simulink model "quadmanipulation"  (R2020a)
settings: Solver=VariableStepAuto  StartTime=0.0  StopTime=30  RelTol=1e-3
values from neighbouring files (symbols this model uses):
  A = [0 0 0 1 0 0 0 0 0 0 0 0 0 0 0 0 ... (first row only)    [quadmanipulation.m]
  B = [0 0 0 0 0 0 ... (first row only)    [quadmanipulation.m]
  B_imp = diag(b_imp)    [quadmanipulation.m]
  G_arm = [(m1+m2)*a1*g*cos(theta1)+m2*g*a2*cos(theta1+theta2) ... (first row only)    [quadmanipulation.m]
  JT = transpose(J)    [quadmanipulation.m]
  K_imp = diag(k_imp)    [quadmanipulation.m]
  M = [m1*a1^2+m2*(a1^2+2*a1*a2*cos(theta2)+a2^2) m2*(a1*a2*cos(theta2)+a2^2) ... (first row only)    [quadmanipulation.m]
  S_arm = [-2*m2*a1*a2*sin(theta2)*theta2_dot -m2*a1*a2*sin(theta2)*theta2_dot ... (first row only)    [quadmanipulation.m]
  theta11 = real(Theta11), theta12 = real(Theta12)    [quadmanipulation.m]
  theta21 = real(Theta21), theta22 = real(Theta22)    [quadmanipulation.m]
undefined symbols (not defined in the file or in its folder): K, theta12, theta22
settings Model: Creator=Dr.Saraf  LastModifiedBy=Dr.Saraf

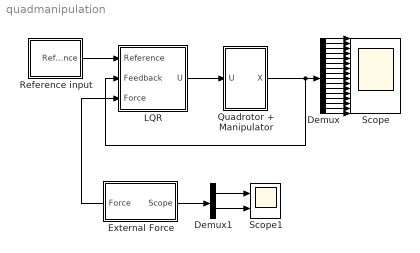
== system quadmanipulation ==
  Demux : Demux  Outputs=16
  Demux1 : Demux  Outputs=2
  External Force : Subsystem
      settings: PortSchema="{\"entries\":[{\"content\":{\"sides\":[{\"content\":{\"connectorIds\":[\"Out2\"]},\"type\":\"ConnectorPlacement.EquallySpacedRectSide\",\"uuid\":\"bc6f37bf-b6c5-4028-b4a4-1f6ac3343290\"},{\"content\":{\"connectorIds\":[\"Out1\"],\"side\":\"RIGHT\"},\"type\":\"ConnectorPlacement.EquallySpacedRectSide\",\"uuid\":\"4c1d6f8d-9a15-4436-8744-0df7d527871c\"},{\"content\":{\"connectorIds\":[],\"side\":\"TOP\"},\"type\":\"ConnectorPlacement.EquallySpacedRectSide\",\"uuid\":\"b806ddfa-c017-4b4f-bf2f-a13602b353a7\"}]},\"type\":\"ConnectorPlacement.EquallySpacedConnector\",\"uuid\":\"efa4b6a4-9e82-4f59-9dc9-02b8956516e8\"}],\"packageUris\":[\"http://schema.mathworks.com/mf0/Connector/19700101\"],\"version\":\"1.0\"}"
  LQR : Subsystem
  Quadrotor + Manipulator : Subsystem
  Reference input : Subsystem
  Scope : Scope  NumInputPorts=16
  Scope1 : Scope  NumInputPorts=2
  wires:
  Quadrotor + Manipulator/1(X) -> LQR/2(Feedback), Demux/1
  Demux/6 -> Scope/6
  Demux/1 -> Scope/1
  Demux/4 -> Scope/4
  LQR/1(U) -> Quadrotor + Manipulator/1(U)
  Demux/3 -> Scope/3
  Demux/5 -> Scope/5
  Demux/2 -> Scope/2
  Reference input/1(Reference) -> LQR/1(Reference)
  Demux/7 -> Scope/7
  Demux/8 -> Scope/8
  Demux/9 -> Scope/9
  Demux/10 -> Scope/10
  Demux/11 -> Scope/11
  Demux/12 -> Scope/12
  Demux/13 -> Scope/13
  Demux/14 -> Scope/14
  Demux/15 -> Scope/15
  Demux/16 -> Scope/16
  External Force/2(Force) -> LQR/3(Force)
  External Force/1(Scope) -> Demux1/1
  Demux1/1 -> Scope1/1
  Demux1/2 -> Scope1/2

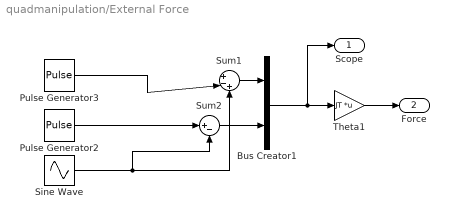
== system quadmanipulation/External Force ==
  Bus Creator1 : BusCreator  Inputs=2
  Pulse Generator2 : DiscretePulseGenerator  PulseType=Time based  Amplitude=4  Period=10  PulseWidth=20
  Pulse Generator3 : DiscretePulseGenerator  PulseType=Time based  Amplitude=5  Period=10  PulseWidth=10  PhaseDelay=4
  Sine Wave : Sin  Amplitude=2  Frequency=2  SampleTime=0
  Sum1 : Sum  Inputs=|+-+
  Sum2 : Sum  Inputs=|+-
  Theta1 : Gain  Gain=JT  Multiplication=Matrix(K*u)
  Scope : Outport
  Force : Outport  Port=2
  wires:
  Bus Creator1/1 -> Scope/1, Theta1/1
  Theta1/1 -> Force/1
  Pulse Generator3/1 -> Sum1/2
  Pulse Generator2/1 -> Sum2/1
  Sine Wave/1 -> Sum2/2, Sum1/3
  Sum2/1 -> Bus Creator1/2
  Sum1/1 -> Bus Creator1/1

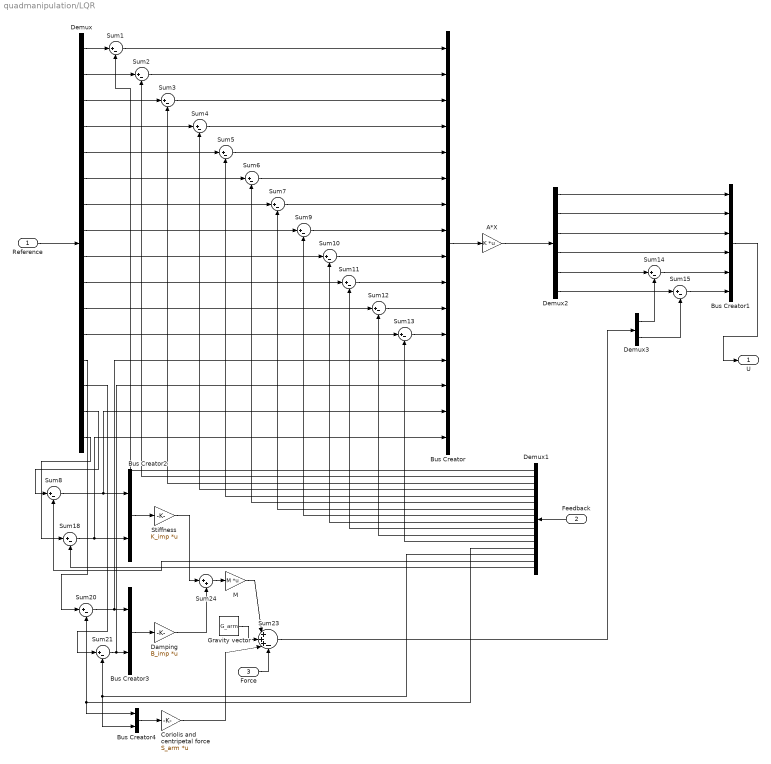
== system quadmanipulation/LQR ==
  Reference : Inport
  Feedback : Inport  Port=2
  Force : Inport  Port=3
  A*X : Gain  Gain=K  Multiplication=Matrix(K*u)
  Bus Creator : BusCreator  Inputs=16
  Bus Creator1 : BusCreator  Inputs=6
  Bus Creator2 : BusCreator  Inputs=2
  Bus Creator3 : BusCreator  Inputs=2
  Bus Creator4 : BusCreator  Inputs=2
  Coriolis and centripetal force : Gain  Gain=S_arm  Multiplication=Matrix(K*u)
  Damping : Gain  Gain=B_imp  Multiplication=Matrix(K*u)
  Demux : Demux  Outputs=16
  Demux1 : Demux  Outputs=16
  Demux2 : Demux  Outputs=6
  Demux3 : Demux  Outputs=2
  Gravity vector : Constant  Value=G_arm  VectorParams1D=off
  M : Gain  Gain=M  Multiplication=Matrix(K*u)
  Stiffness : Gain  Gain=K_imp  Multiplication=Matrix(K*u)
  Sum{1..15,18,20..21} (18 alike) : Sum  Inputs=|+-
  Sum23 : Sum  Inputs=|+++-
  Sum24 : Sum  Inputs=|++
  U : Outport
  wires:
  Bus Creator/1 -> A*X/1
  Sum2/1 -> Bus Creator/2
  Sum6/1 -> Bus Creator/6
  Sum3/1 -> Bus Creator/3
  Sum5/1 -> Bus Creator/5
  Sum4/1 -> Bus Creator/4
  Demux/6 -> Sum6/1
  Demux1/5 -> Sum5/2
  Demux1/3 -> Sum3/2
  Demux1/2 -> Sum2/2
  Demux/1 -> Sum1/1
  Sum1/1 -> Bus Creator/1
  Demux1/4 -> Sum4/2
  Demux1/6 -> Sum6/2
  Demux/2 -> Sum2/1
  Demux1/1 -> Sum1/2
  Feedback/1 -> Demux1/1
  Demux/3 -> Sum3/1
  Demux/5 -> Sum5/1
  Demux/4 -> Sum4/1
  Reference/1 -> Demux/1
  Sum13/1 -> Bus Creator/12
  Demux/12 -> Sum13/1
  Sum12/1 -> Bus Creator/11
  Demux/11 -> Sum12/1
  Sum11/1 -> Bus Creator/10
  Demux/10 -> Sum11/1
  Sum10/1 -> Bus Creator/9
  Demux/9 -> Sum10/1
  Sum9/1 -> Bus Creator/8
  Sum7/1 -> Bus Creator/7
  Demux/7 -> Sum7/1
  Demux/8 -> Sum9/1
  Demux1/7 -> Sum7/2
  Demux1/8 -> Sum9/2
  Demux1/9 -> Sum10/2
  Demux1/10 -> Sum11/2
  Demux1/11 -> Sum12/2
  Demux1/12 -> Sum13/2
  Demux/14 -> Sum21/1
  Bus Creator3/1 -> Damping/1
  Coriolis and centripetal force/1 -> Sum23/3
  Sum24/1 -> M/1
  Demux/15 -> Sum8/1
  Demux1/15 -> Sum8/2
  Sum18/1 -> Bus Creator/16, Bus Creator2/2
  Demux1/16 -> Sum18/2
  Damping/1 -> Sum24/2
  Demux/13 -> Sum20/1
  Sum20/1 -> Bus Creator/13, Bus Creator3/1
  Demux/16 -> Sum18/1
  Sum21/1 -> Bus Creator/14, Bus Creator3/2
  Force/1 -> Sum23/4
  Bus Creator4/1 -> Coriolis and centripetal force/1
  M/1 -> Sum23/1
  Bus Creator2/1 -> Stiffness/1
  Gravity vector/1 -> Sum23/2
  Stiffness/1 -> Sum24/1
  Sum8/1 -> Bus Creator/15, Bus Creator2/1
  Demux1/13 -> Bus Creator4/1, Sum20/2
  Demux1/14 -> Bus Creator4/2, Sum21/2
  Bus Creator1/1 -> U/1
  A*X/1 -> Demux2/1
  Sum23/1 -> Demux3/1
  Sum15/1 -> Bus Creator1/6
  Demux2/1 -> Bus Creator1/1
  Demux2/2 -> Bus Creator1/2
  Demux2/3 -> Bus Creator1/3
  Demux2/4 -> Bus Creator1/4
  Demux2/5 -> Sum14/1
  Sum14/1 -> Bus Creator1/5
  Demux2/6 -> Sum15/1
  Demux3/1 -> Sum14/2
  Demux3/2 -> Sum15/2

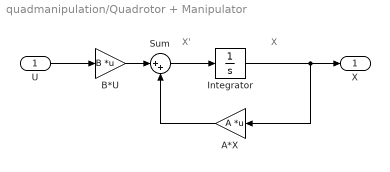
== system quadmanipulation/Quadrotor + Manipulator ==
  note: X'
  note: X
  U : Inport
  A*X : Gain  Gain=A  Multiplication=Matrix(K*u)
  B*U : Gain  Gain=B  Multiplication=Matrix(K*u)
  Integrator : Integrator  InitialCondition=[0,0,0,0,0,0,0,0,0,0,0,0,0,0,theta11, theta12]
  Sum : Sum  Inputs=|++
  X : Outport
  wires:
  Integrator/1 -> X/1, A*X/1
  Sum/1 -> Integrator/1
  U/1 -> B*U/1
  A*X/1 -> Sum/2
  B*U/1 -> Sum/1

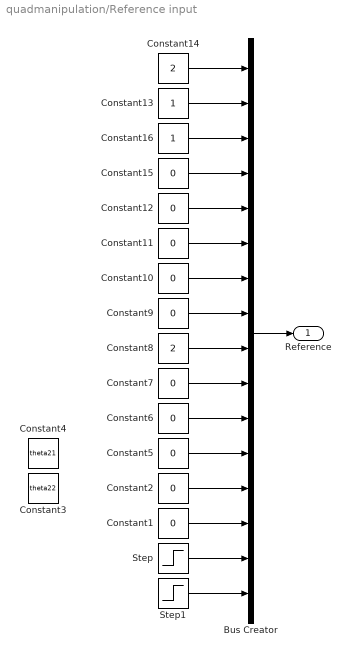
== system quadmanipulation/Reference input ==
  Bus Creator : BusCreator  Inputs=16
  Constant{1..2,5..7,9..12,15} (10 alike) : Constant  Value=0
  Constant13 : Constant
  Constant14 : Constant  Value=2
  Constant16 : Constant
  Constant3 : Constant  Value=theta22
  Constant4 : Constant  Value=theta21
  Constant8 : Constant  Value=2
  Step : Step  Time=5  Before=theta11  After=theta21  SampleTime=0
  Step1 : Step  Time=5  Before=theta12  After=theta22  SampleTime=0
  Reference : Outport
  wires:
  Bus Creator/1 -> Reference/1
  Constant2/1 -> Bus Creator/13
  Constant1/1 -> Bus Creator/14
  Step/1 -> Bus Creator/15
  Constant5/1 -> Bus Creator/12
  Constant6/1 -> Bus Creator/11
  Constant7/1 -> Bus Creator/10
  Constant8/1 -> Bus Creator/9
  Constant9/1 -> Bus Creator/8
  Constant10/1 -> Bus Creator/7
  Constant11/1 -> Bus Creator/6
  Constant12/1 -> Bus Creator/5
  Constant13/1 -> Bus Creator/2
  Constant14/1 -> Bus Creator/1
  Constant15/1 -> Bus Creator/4
  Constant16/1 -> Bus Creator/3
  Step1/1 -> Bus Creator/16
